simulink subsystem "H175_cathode"  (R2022b)
settings: Solver=VariableStepAuto  StartTime=0.0  StopTime=10.0  RelTol=1e-3
libraries: fl_lib x88, nesl_utility x73, SimscapeFluids_lib x10, slpidlib x2, BraytonCycle_lib x2
(part 4 of 4)

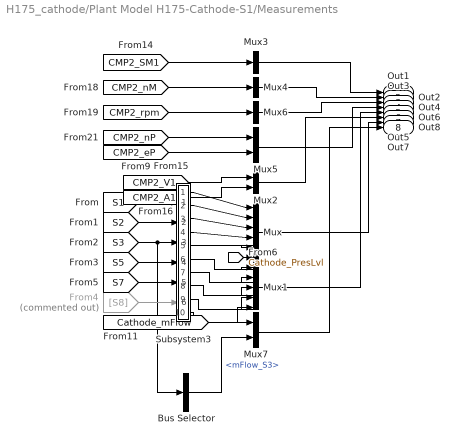
== system H175_cathode/Plant Model H175-Cathode-S1/Measurements ==
  Bus Selector : BusSelector  OutputSignals=mFlow_S3
  From4 : From  Commented=on  GotoTag=S8
  Mux : Mux  Inputs=6
  Mux1 : Mux  Inputs=5
  Mux2 : Mux  Inputs=2
  Mux3 : Mux  Inputs=1
  Mux4 : Mux  Inputs=1
  Mux5 : Mux  Inputs=2
  Mux6 : Mux  Inputs=1
  Mux7 : Mux  Inputs=2
  Subsystem3 : Subsystem
  Out1 : Outport
  Out2 : Outport  Port=2
  Out3 : Outport  Port=3
  Out4 : Outport  Port=4
  Out5 : Outport  Port=5
  Out6 : Outport  Port=6
  Out7 : Outport  Port=7
  Out8 : Outport  Port=8
  wires:
  Mux4/1 -> Out2/1
  Mux6/1 -> Out3/1
  Mux/1 -> Out7/1
  Subsystem3/6(<aTemp_S1>) -> Mux1/1
  Subsystem3/4(<aPres_S5>) -> Mux/4
  [CMP2_rpm] -> Mux6/1
  Subsystem3/3(<aPres_S3>) -> Mux/3
  Subsystem3/9(<aTemp_S5>) -> Mux1/4
  [S3] -> Subsystem3/3(In5), Bus Selector/1
  Subsystem3/8(<aTemp_S3>) -> Mux1/3
  Subsystem3/5(<aPres_S7>) -> Mux/5
  [S5] -> Subsystem3/4(In6)
  [CMP2_nP] -> Mux5/1
  Mux1/1 -> Out5/1
  Subsystem3/2(<aPres_S2>) -> Mux/2
  Mux7/1 -> Out8/1
  [CMP2_V1] -> Mux2/1
  From4/1 -> Subsystem3/6(In8)
  [S2] -> Subsystem3/2(In4)
  [CMP2_nM] -> Mux4/1
  Subsystem3/1(<aPres_S1>) -> Mux/1
  Bus Selector/1 -> Mux7/2  "<mFlow_S3>"
  Mux5/1 -> Out4/1
  Mux2/1 -> Out6/1
  [CMP2_A1] -> Mux2/2
  [CMP2_SM1] -> Mux3/1
  Subsystem3/7(<aTemp_S2>) -> Mux1/2
  Subsystem3/10(<aTemp_S7>) -> Mux1/5
  [S7] -> Subsystem3/5(In7)
  [Cathode_mFlow] -> Mux7/1
  [CMP2_eP] -> Mux5/2
  Mux3/1 -> Out1/1
  [S1] -> Subsystem3/1(In3)
  [Cathode_PresLvl] -> Mux/6

== system H175_cathode/Plant Model H175-Cathode-S1/Outlet ==
  Controlled Reservoir (G)1 : fl_lib/Gas/Elements/Controlled Reservoir (G)  area_A=0.002 m^2
      settings: InternalSimscapePortConfiguration="{\"Bottom\":[],\"Left\":[{\"id\":\"A\",\"label\":\"A\",\"type\":\"foundation.gas.gas\"}],\"Right\":[{\"id\":\"T_in\",\"label\":\"T\",\"type\":\"input\"},{\"id\":\"p_in\",\"label\":\"P\",\"type\":\"input\"}],\"Top\":[]}"
  Flow Resistance (G) : fl_lib/Gas/Elements/Flow Resistance (G)  delta_p_nominal=.15 bar  mdot_nominal=.3 kg/s  rho_nominal=2.1 kg/m^3  area=0.01 m^2  laminar_fraction=1e-3
      settings: InternalSimscapePortConfiguration="{\"Bottom\":[],\"Left\":[{\"id\":\"A\",\"label\":\"A\",\"type\":\"foundation.gas.gas\"}],\"Right\":[{\"id\":\"B\",\"label\":\"B\",\"type\":\"foundation.gas.gas\"}],\"Top\":[]}"
  Conn1 : PMIOPort  Side=Left
  Conn2 : PMIOPort  Port=2  Side=Left
  Conn3 : PMIOPort  Port=3  Side=Right
  connections:
  Flow Resistance (G)/RConn1 -- Conn3/RConn1
  Controlled Reservoir (G)1/RConn1 -- Conn2/RConn1
  Controlled Reservoir (G)1/LConn1 -- Flow Resistance (G)/LConn1
  Controlled Reservoir (G)1/RConn2 -- Conn1/RConn1

== system H175_cathode/Plant Model H175-Cathode-S1/S1 ==
  Absolute Reference (G) : fl_lib/Gas/Elements/Absolute Reference (G)
      settings: InternalSimscapePortConfiguration="{\"Bottom\":[],\"Left\":[{\"id\":\"A\",\"label\":\"\",\"type\":\"foundation.gas.gas\"}],\"Right\":[],\"Top\":[]}"
  Bus Creator : BusCreator  Inputs=3
  Mass & Energy Flow Rate Sensor (G) : fl_lib/Gas/Sensors/Mass & Energy Flow Rate Sensor (G)
      settings: InternalSimscapePortConfiguration="{\"Bottom\":[],\"Left\":[{\"id\":\"A\",\"label\":\"A\",\"type\":\"foundation.gas.gas\"}],\"Right\":[{\"id\":\"B\",\"label\":\"B\",\"type\":\"foundation.gas.gas\"},{\"id\":\"M\",\"label\":\"M\",\"type\":\"output\"},{\"id\":\"PHI\",\"label\":\"Phi\",\"type\":\"output\"}],\"Top\":[]}"
  Pressure & Temperature Sensor (G)4 : fl_lib/Gas/Sensors/Pressure & Temperature Sensor (G)
      settings: InternalSimscapePortConfiguration="{\"Bottom\":[],\"Left\":[{\"id\":\"A\",\"label\":\"A\",\"type\":\"foundation.gas.gas\"}],\"Right\":[{\"id\":\"B\",\"label\":\"B\",\"type\":\"foundation.gas.gas\"},{\"id\":\"P\",\"label\":\"P\",\"type\":\"output\"},{\"id\":\"T\",\"label\":\"T\",\"type\":\"output\"}],\"Top\":[]}"
  aPres_S1 : nesl_utility/PS-Simulink Converter  PhysicalDomain=network_engine_domain  SubClassName=ps_output  LeftPortType=input  RightPortType=output  PseudoPeriodic=off  Frequencies=[]  VectorFormat=inherit  Unit=inherit  AffineConversion=off
  aTemp_S1 : nesl_utility/PS-Simulink Converter  PhysicalDomain=network_engine_domain  SubClassName=ps_output  LeftPortType=input  RightPortType=output  PseudoPeriodic=off  Frequencies=[]  VectorFormat=inherit  Unit=inherit  AffineConversion=off
  aTemp_S2 : nesl_utility/PS-Simulink Converter  PhysicalDomain=network_engine_domain  SubClassName=ps_output  LeftPortType=input  RightPortType=output  PseudoPeriodic=off  Frequencies=[]  VectorFormat=inherit  Unit=inherit  AffineConversion=off
  Conn1 : PMIOPort  Side=Left
  Conn2 : PMIOPort  Port=2  Side=Right
  Out1 : Outport
  wires:
  aTemp_S2/1 -> Bus Creator/3  "mFlow_S1"
  Bus Creator/1 -> Out1/1
  aPres_S1/1 -> Bus Creator/1  "aPres_S1"
  aTemp_S1/1 -> Bus Creator/2  "aTemp_S1"
  connections:
  Mass & Energy Flow Rate Sensor (G)/RConn1 -- Conn2/RConn1
  Mass & Energy Flow Rate Sensor (G)/RConn2 -- aTemp_S2/LConn1
  Conn1/RConn1 -- Pressure & Temperature Sensor (G)4/LConn1 -- Mass & Energy Flow Rate Sensor (G)/LConn1
  aTemp_S1/LConn1 -- Pressure & Temperature Sensor (G)4/RConn3
  aPres_S1/LConn1 -- Pressure & Temperature Sensor (G)4/RConn2
  Absolute Reference (G)/LConn1 -- Pressure & Temperature Sensor (G)4/RConn1

== system H175_cathode/Plant Model H175-Cathode-S1/S2 ==
  Absolute Reference (G) : fl_lib/Gas/Elements/Absolute Reference (G)
      settings: InternalSimscapePortConfiguration="{\"Bottom\":[],\"Left\":[{\"id\":\"A\",\"label\":\"\",\"type\":\"foundation.gas.gas\"}],\"Right\":[],\"Top\":[]}"
  Bus Creator : BusCreator  Inputs=3
  Mass & Energy Flow Rate Sensor (G) : fl_lib/Gas/Sensors/Mass & Energy Flow Rate Sensor (G)
      settings: InternalSimscapePortConfiguration="{\"Bottom\":[],\"Left\":[{\"id\":\"A\",\"label\":\"A\",\"type\":\"foundation.gas.gas\"}],\"Right\":[{\"id\":\"B\",\"label\":\"B\",\"type\":\"foundation.gas.gas\"},{\"id\":\"M\",\"label\":\"M\",\"type\":\"output\"},{\"id\":\"PHI\",\"label\":\"Phi\",\"type\":\"output\"}],\"Top\":[]}"
  Pressure & Temperature Sensor (G)4 : fl_lib/Gas/Sensors/Pressure & Temperature Sensor (G)
      settings: InternalSimscapePortConfiguration="{\"Bottom\":[],\"Left\":[{\"id\":\"A\",\"label\":\"A\",\"type\":\"foundation.gas.gas\"}],\"Right\":[{\"id\":\"B\",\"label\":\"B\",\"type\":\"foundation.gas.gas\"},{\"id\":\"P\",\"label\":\"P\",\"type\":\"output\"},{\"id\":\"T\",\"label\":\"T\",\"type\":\"output\"}],\"Top\":[]}"
  aPres_S1 : nesl_utility/PS-Simulink Converter  PhysicalDomain=network_engine_domain  SubClassName=ps_output  LeftPortType=input  RightPortType=output  PseudoPeriodic=off  Frequencies=[]  VectorFormat=inherit  Unit=inherit  AffineConversion=off
  aTemp_S1 : nesl_utility/PS-Simulink Converter  PhysicalDomain=network_engine_domain  SubClassName=ps_output  LeftPortType=input  RightPortType=output  PseudoPeriodic=off  Frequencies=[]  VectorFormat=inherit  Unit=degC  AffineConversion=off
  mFlow_S2 : nesl_utility/PS-Simulink Converter  PhysicalDomain=network_engine_domain  SubClassName=ps_output  LeftPortType=input  RightPortType=output  PseudoPeriodic=off  Frequencies=[]  VectorFormat=inherit  Unit=inherit  AffineConversion=off
  Conn1 : PMIOPort  Side=Left
  Conn2 : PMIOPort  Port=2  Side=Right
  Out1 : Outport
  wires:
  mFlow_S2/1 -> Bus Creator/3  "mFlow_S2"
  aTemp_S1/1 -> Bus Creator/2  "aTemp_S2"
  aPres_S1/1 -> Bus Creator/1  "aPres_S2"
  Bus Creator/1 -> Out1/1
  connections:
  Mass & Energy Flow Rate Sensor (G)/RConn2 -- mFlow_S2/LConn1
  Mass & Energy Flow Rate Sensor (G)/RConn1 -- Conn2/RConn1
  aTemp_S1/LConn1 -- Pressure & Temperature Sensor (G)4/RConn3
  aPres_S1/LConn1 -- Pressure & Temperature Sensor (G)4/RConn2
  Absolute Reference (G)/LConn1 -- Pressure & Temperature Sensor (G)4/RConn1
  Conn1/RConn1 -- Mass & Energy Flow Rate Sensor (G)/LConn1 -- Pressure & Temperature Sensor (G)4/LConn1

== system H175_cathode/Plant Model H175-Cathode-S1/S3 ==
  Absolute Reference (G) : fl_lib/Gas/Elements/Absolute Reference (G)
      settings: InternalSimscapePortConfiguration="{\"Bottom\":[],\"Left\":[{\"id\":\"A\",\"label\":\"\",\"type\":\"foundation.gas.gas\"}],\"Right\":[],\"Top\":[]}"
  Bus Creator : BusCreator  Inputs=3
  Mass & Energy Flow Rate Sensor (G) : fl_lib/Gas/Sensors/Mass & Energy Flow Rate Sensor (G)
      settings: InternalSimscapePortConfiguration="{\"Bottom\":[],\"Left\":[{\"id\":\"A\",\"label\":\"A\",\"type\":\"foundation.gas.gas\"}],\"Right\":[{\"id\":\"B\",\"label\":\"B\",\"type\":\"foundation.gas.gas\"},{\"id\":\"M\",\"label\":\"M\",\"type\":\"output\"},{\"id\":\"PHI\",\"label\":\"Phi\",\"type\":\"output\"}],\"Top\":[]}"
  Pressure & Temperature Sensor (G)4 : fl_lib/Gas/Sensors/Pressure & Temperature Sensor (G)
      settings: InternalSimscapePortConfiguration="{\"Bottom\":[],\"Left\":[{\"id\":\"A\",\"label\":\"A\",\"type\":\"foundation.gas.gas\"}],\"Right\":[{\"id\":\"B\",\"label\":\"B\",\"type\":\"foundation.gas.gas\"},{\"id\":\"P\",\"label\":\"P\",\"type\":\"output\"},{\"id\":\"T\",\"label\":\"T\",\"type\":\"output\"}],\"Top\":[]}"
  aPres_S1 : nesl_utility/PS-Simulink Converter  PhysicalDomain=network_engine_domain  SubClassName=ps_output  LeftPortType=input  RightPortType=output  PseudoPeriodic=off  Frequencies=[]  VectorFormat=inherit  Unit=inherit  AffineConversion=off
  aPres_S2 : nesl_utility/PS-Simulink Converter  PhysicalDomain=network_engine_domain  SubClassName=ps_output  LeftPortType=input  RightPortType=output  PseudoPeriodic=off  Frequencies=[]  VectorFormat=inherit  Unit=inherit  AffineConversion=off
  aTemp_S1 : nesl_utility/PS-Simulink Converter  PhysicalDomain=network_engine_domain  SubClassName=ps_output  LeftPortType=input  RightPortType=output  PseudoPeriodic=off  Frequencies=[]  VectorFormat=inherit  Unit=degC  AffineConversion=off
  Conn2 : PMIOPort  Side=Left
  Conn1 : PMIOPort  Port=2  Side=Right
  Out1 : Outport
  wires:
  aPres_S2/1 -> Bus Creator/3  "mFlow_S3"
  Bus Creator/1 -> Out1/1
  aPres_S1/1 -> Bus Creator/1  "aPres_S3"
  aTemp_S1/1 -> Bus Creator/2  "aTemp_S3"
  connections:
  Mass & Energy Flow Rate Sensor (G)/RConn2 -- aPres_S2/LConn1
  Conn1/RConn1 -- Mass & Energy Flow Rate Sensor (G)/LConn1 -- Pressure & Temperature Sensor (G)4/LConn1
  aTemp_S1/LConn1 -- Pressure & Temperature Sensor (G)4/RConn3
  aPres_S1/LConn1 -- Pressure & Temperature Sensor (G)4/RConn2
  Absolute Reference (G)/LConn1 -- Pressure & Temperature Sensor (G)4/RConn1
  Mass & Energy Flow Rate Sensor (G)/RConn1 -- Conn2/RConn1

== system H175_cathode/Plant Model H175-Cathode-S1/S5 ==
  Absolute Reference (G) : fl_lib/Gas/Elements/Absolute Reference (G)
      settings: InternalSimscapePortConfiguration="{\"Bottom\":[],\"Left\":[{\"id\":\"A\",\"label\":\"\",\"type\":\"foundation.gas.gas\"}],\"Right\":[],\"Top\":[]}"
  Bus Creator : BusCreator  Inputs=2
  Pressure & Temperature Sensor (G)4 : fl_lib/Gas/Sensors/Pressure & Temperature Sensor (G)
      settings: InternalSimscapePortConfiguration="{\"Bottom\":[],\"Left\":[{\"id\":\"A\",\"label\":\"A\",\"type\":\"foundation.gas.gas\"}],\"Right\":[{\"id\":\"B\",\"label\":\"B\",\"type\":\"foundation.gas.gas\"},{\"id\":\"P\",\"label\":\"P\",\"type\":\"output\"},{\"id\":\"T\",\"label\":\"T\",\"type\":\"output\"}],\"Top\":[]}"
  aPres_S1 : nesl_utility/PS-Simulink Converter  PhysicalDomain=network_engine_domain  SubClassName=ps_output  LeftPortType=input  RightPortType=output  PseudoPeriodic=off  Frequencies=[]  VectorFormat=inherit  Unit=inherit  AffineConversion=off
  aTemp_S1 : nesl_utility/PS-Simulink Converter  PhysicalDomain=network_engine_domain  SubClassName=ps_output  LeftPortType=input  RightPortType=output  PseudoPeriodic=off  Frequencies=[]  VectorFormat=inherit  Unit=degC  AffineConversion=off
  Conn1 : PMIOPort  Side=Left
  Conn2 : PMIOPort  Port=2  Side=Right
  Out1 : Outport
  wires:
  aTemp_S1/1 -> Bus Creator/2  "aTemp_S5"
  aPres_S1/1 -> Bus Creator/1  "aPres_S5"
  Bus Creator/1 -> Out1/1
  connections:
  aTemp_S1/LConn1 -- Pressure & Temperature Sensor (G)4/RConn3
  aPres_S1/LConn1 -- Pressure & Temperature Sensor (G)4/RConn2
  Absolute Reference (G)/LConn1 -- Pressure & Temperature Sensor (G)4/RConn1
  Conn2/RConn1 -- Conn1/RConn1 -- Pressure & Temperature Sensor (G)4/LConn1

== system H175_cathode/Plant Model H175-Cathode-S1/S7 ==
  Absolute Reference (G) : fl_lib/Gas/Elements/Absolute Reference (G)
      settings: InternalSimscapePortConfiguration="{\"Bottom\":[],\"Left\":[{\"id\":\"A\",\"label\":\"\",\"type\":\"foundation.gas.gas\"}],\"Right\":[],\"Top\":[]}"
  Bus Creator : BusCreator  Inputs=3
  Mass & Energy Flow Rate Sensor (G) : fl_lib/Gas/Sensors/Mass & Energy Flow Rate Sensor (G)
      settings: InternalSimscapePortConfiguration="{\"Bottom\":[],\"Left\":[{\"id\":\"A\",\"label\":\"A\",\"type\":\"foundation.gas.gas\"}],\"Right\":[{\"id\":\"B\",\"label\":\"B\",\"type\":\"foundation.gas.gas\"},{\"id\":\"M\",\"label\":\"M\",\"type\":\"output\"},{\"id\":\"PHI\",\"label\":\"Phi\",\"type\":\"output\"}],\"Top\":[]}"
  Pressure & Temperature Sensor (G)4 : fl_lib/Gas/Sensors/Pressure & Temperature Sensor (G)
      settings: InternalSimscapePortConfiguration="{\"Bottom\":[],\"Left\":[{\"id\":\"A\",\"label\":\"A\",\"type\":\"foundation.gas.gas\"}],\"Right\":[{\"id\":\"B\",\"label\":\"B\",\"type\":\"foundation.gas.gas\"},{\"id\":\"P\",\"label\":\"P\",\"type\":\"output\"},{\"id\":\"T\",\"label\":\"T\",\"type\":\"output\"}],\"Top\":[]}"
  aPres_S1 : nesl_utility/PS-Simulink Converter  PhysicalDomain=network_engine_domain  SubClassName=ps_output  LeftPortType=input  RightPortType=output  PseudoPeriodic=off  Frequencies=[]  VectorFormat=inherit  Unit=inherit  AffineConversion=off
  aTemp_S1 : nesl_utility/PS-Simulink Converter  PhysicalDomain=network_engine_domain  SubClassName=ps_output  LeftPortType=input  RightPortType=output  PseudoPeriodic=off  Frequencies=[]  VectorFormat=inherit  Unit=degC  AffineConversion=off
  mFlow_S7 : nesl_utility/PS-Simulink Converter  PhysicalDomain=network_engine_domain  SubClassName=ps_output  LeftPortType=input  RightPortType=output  PseudoPeriodic=off  Frequencies=[]  VectorFormat=inherit  Unit=kg/s  AffineConversion=off
  Conn1 : PMIOPort  Side=Left
  Conn2 : PMIOPort  Port=2  Side=Right
  Out1 : Outport
  wires:
  mFlow_S7/1 -> Bus Creator/3  "mFlow_S7"
  Bus Creator/1 -> Out1/1
  aPres_S1/1 -> Bus Creator/1  "aPres_S7"
  aTemp_S1/1 -> Bus Creator/2  "aTemp_S7"
  connections:
  Conn2/RConn1 -- Mass & Energy Flow Rate Sensor (G)/RConn1
  Mass & Energy Flow Rate Sensor (G)/RConn2 -- mFlow_S7/LConn1
  aTemp_S1/LConn1 -- Pressure & Temperature Sensor (G)4/RConn3
  aPres_S1/LConn1 -- Pressure & Temperature Sensor (G)4/RConn2
  Absolute Reference (G)/LConn1 -- Pressure & Temperature Sensor (G)4/RConn1
  Mass & Energy Flow Rate Sensor (G)/LConn1 -- Pressure & Temperature Sensor (G)4/LConn1 -- Conn1/RConn1

== system H175_cathode/Plant Model H175-Cathode-S1/Subsystem ==
  Bus Selector : BusSelector  OutputSignals=aPres_S1,aTemp_S1
  Bus Selector1 : BusSelector  OutputSignals=aPres_S2
  Bus Selector2 : BusSelector  OutputSignals=aTemp_S3,aPres_S3,mFlow_S3
  <aPres_S1> : Outport
  <aTemp_S1> : Outport  Port=2
  <mFlow_S2> : Outport  Port=3
  <aPres_S2> : Outport  Port=4
  <aTemp_S3> : Outport  Port=5
  <aPres_S3> : Outport  Port=6
  wires:
  Bus Selector2/3 -> <mFlow_S2>/1  "<mFlow_S3>"
  Bus Selector2/2 -> <aPres_S3>/1  "<aPres_S3>"
  Bus Selector/2 -> <aTemp_S1>/1  "<aTemp_S1>"
  Bus Selector1/1 -> <aPres_S2>/1  "<aPres_S2>"
  Bus Selector2/1 -> <aTemp_S3>/1  "<aTemp_S3>"
  [S3] -> Bus Selector2/1
  [S1] -> Bus Selector/1
  Bus Selector/1 -> <aPres_S1>/1  "<aPres_S1>"
  [S2] -> Bus Selector1/1

== system H175_cathode/Plant Model H175-Cathode-S1/VL6513 ==
  input0 : Inport
  Display : Display
  Orifice (G) : SimscapeFluids_lib/Gas/Valves & Orifices/Orifice (G)  orifice_type=foundation.enum.constant_variable.variable  orifice_parameterization=fluids.gas.valves_orifices.enum.OrificeParameterization.Area  opening_characteristic=fluids.gas.valves_orifices.enum.OpeningCharacteristics.Tabulated  Cv_constant=4  Cv_max=169.7  L_Cv_TLU=0 : 0.2 : 1  Cv_TLU=[1e-06, .8, 1.6, 2.4, 3.2, 4]  xT_Cv=0.7  Kv_constant=3.6  Kv_max=10  L_Kv_TLU=0 : 0.2 : 1  Kv_TLU=[1e-06, .72, 1.44, 2.16, 2.88, 3.6]  xT_Kv=0.7  C_constant=12 l/(bar*s)  B_crit_constant=0.3  C_max=12 l/(bar*s)  B_crit_linear=0.3  L_C_TLU=0 : 0.2 : 1  C_TLU=[1e-05, 2.4, 4.8, 7.2, 9.6, 12] l/(bar*s)  B_crit_TLU=0.3 * ones(1, 6)  m=0.5  T_ref_C=293.15 K  rho_ref_C=1.185 kg/m^3  orifice_area_constant=1e-4 m^2  orifice_area_max=0.00145 m^2  L_orifice_area_TLU=[0.00889,0.15555,0.26,0.36444,0.46889,0.57222,0.676666,0.7811,0.88555,0.9277]  orifice_area_TLU=[0.000258,0.00146,0.001674,0.0018,0.00189,0.001946,0.0019564,0.001995,0.001999,0.002] m^2  Cd=.8  leakage_fraction=1e-6  smoothing_factor=0.02  B_lam=0.999  area=0.0021 m^2  mdot_A_specify=off  mdot_A_priority=None  mdot_A=0 kg/s  mdot_A_nominal_specify=off  mdot_A_nominal_unit=kg/s  mdot_A_nominal_value=1  mdot_B_specify=off  mdot_B_priority=None  mdot_B=0 kg/s  mdot_B_nominal_specify=off  mdot_B_nominal_unit=kg/s  mdot_B_nominal_value=1  Phi_A_specify=off  Phi_A_priority=None  Phi_A=0 kW  Phi_A_nominal_specify=off  Phi_A_nominal_unit=kW  Phi_A_nominal_value=1  Phi_B_specify=off  Phi_B_priority=None  Phi_B=0 kW  Phi_B_nominal_specify=off  Phi_B_nominal_unit=kW  Phi_B_nominal_value=1
      settings: InternalSimscapePortConfiguration="{\"Bottom\":[],\"Left\":[{\"id\":\"A\",\"label\":\"A\",\"type\":\"foundation.gas.gas\"},{\"id\":\"L\",\"label\":\"L\",\"type\":\"input\"}],\"Right\":[{\"id\":\"B\",\"label\":\"B\",\"type\":\"foundation.gas.gas\"}],\"Top\":[]}"
  Simulink-PS Converter3 : nesl_utility/Simulink-PS Converter  PhysicalDomain=network_engine_domain  SubClassName=ps_input  LeftPortType=input  RightPortType=output  PseudoPeriodic=off  Frequencies=[]  NoiseDistribution=none  NoiseParameters=[]  Unit=1  AffineConversion=off  FilteringAndDerivatives=filter  SimscapeFilterOrder=1  InputFilterTimeConstant=0.001  UdotUserProvided=0
  Conn1 : PMIOPort  Side=Left
  Conn2 : PMIOPort  Port=2  Side=Right
  wires:
  input0/1 -> Simulink-PS Converter3/1, Display/1
  connections:
  Orifice (G)/LConn1 -- Conn2/RConn1
  Conn1/RConn1 -- Orifice (G)/RConn1
  Simulink-PS Converter3/RConn1 -- Orifice (G)/LConn2

== system H175_cathode/Humidifier/Cathode Humidifier1/Proportional Control ==
  RH_set : Inport
  RH_meas : Inport  Port=2
  Gain : Gain  Commented=on  Gain=0.1
  PID Controller : slpidlib/PID Controller  Controller=PI  Form=Parallel  TimeDomain=Continuous-time  UseExternalTs=off  SampleTime=-1  IntegratorMethod=Forward Euler  FilterMethod=Forward Euler  ControllerParametersSource=internal  P=1  I=1  UseKiTs=off  D=0  N=100  UseFilter=on  TunerSelectOption=Transfer Function Based (PID Tuner App)  InitialConditionSource=internal  InitialConditionForIntegrator=0  InitialConditionForFilter=0  DifferentiatorICPrevScaledInput=0  ExternalReset=none  TrackingMode=off  Kt=1  LimitOutput=off  SatLimitsSource=internal  UpperSaturationLimit=inf  LowerSaturationLimit=-inf  LinearizeAsGain=on  AntiWindupMode=none  Kb=1  LimitIntegrator=off  UpperIntegratorSaturationLimit=inf  LowerIntegratorSaturationLimit=-inf  POutMin=[]  POutMax=[]  IOutMin=[]  IOutMax=[]  DOutMin=[]  DOutMax=[]  NOutMin=[]  NOutMax=[]  SumOutMin=[]  SumOutMax=[]  SaturationOutMin=[]  SaturationOutMax=[]  PParamMin=[]  PParamMax=[]  IParamMin=[]  IParamMax=[]  DParamMin=[]  DParamMax=[]  NParamMin=[]  NParamMax=[]  KbParamMin=[]  KbParamMax=[]  KtParamMin=[]  KtParamMax=[]  KbOutMin=[]  KbOutMax=[]  KtOutMin=[]  KtOutMax=[]  IntegratorOutMin=[]  IntegratorOutMax=[]  FilterOutMin=[]  FilterOutMax=[]  SumI1OutMin=[]  SumI1OutMax=[]  SumI2OutMin=[]  SumI2OutMax=[]  SumI3OutMin=[]  SumI3OutMax=[]  SumI4OutMin=[]  SumI4OutMax=[]  SumDOutMin=[]  SumDOutMax=[]  DifferentiatorOutMin=[]  DifferentiatorOutMax=[]  FilterDiffOutCoefMin=[]  FilterDiffOutCoefMax=[]  ReciprocalOutMin=[]  ReciprocalOutMax=[]  SumDenOutMin=[]  SumDenOutMax=[]  SumNumOutMin=[]  SumNumOutMax=[]  DivideOutMin=[]  DivideOutMax=[]  UdiffTsProdOutMin=[]  UdiffTsProdOutMax=[]  NTsProdOutMin=[]  NTsProdOutMax=[]  UintegralTsProdOutMin=[]  UintegralTsProdOutMax=[]  UngainTsProdOutMin=[]  UngainTsProdOutMax=[]  ClampingZeroOutDataTypeStr=Inherit: Inherit via back propagation  ClampingZeroOutMin=[]  ClampingZeroOutMax=[]  FilterDenConstantOutDataTypeStr=Inherit: Inherit via back propagation  FilterDenConstantOutMin=[]  FilterDenConstantOutMax=[]  PCopyOutDataTypeStr=Inherit: Inherit via back propagation  PCopyOutMin=[]  PCopyOutMax=[]  NCopyOutDataTypeStr=Inherit: Inherit via back propagation  NCopyOutMin=[]  NCopyOutMax=[]  IntegratorContinuousStateAttributes=''  IntegratorStateMustResolveToSignalObject=off  IntegratorRTWStateStorageClass=Auto  FilterContinuousStateAttributes=''  FilterStateMustResolveToSignalObject=off  FilterRTWStateStorageClass=Auto  ParallelPVariant=InternalParameters  IdealPVariant=Disabled  IVariant=InternalParameters  DVariant=Disabled  IntegratorVariant=Continuous  SatVariant=Disabled  AWVariant=Passthrough  PCopyVariant=Disabled  TRVariant=Disabled  FdbkBlocksVariant=Forward  IdealPFdbkVariant=Disabled  SatFdbkVariant=Disabled  DerivativeFilterVariant=Disabled  NVariant=Disabled  NCopyVariant=Disabled_SignalSpec  FilterICVariant=Disabled  IntegratorICVariant=InternalICs  ExternalResetVariant=Disabled  TRSumVariant=Passthrough  SumFdbkVariant=Disabled  SumVariant=Sum_PI  TsampFilterVariant=InternalTs  TsampNgainVariant=Passthrough  TsampIntegralVariant=Passthrough  ExternalSaturationOutDataTypeStr=Inherit: Same as second input
  Saturation : Saturate  Commented=on  UpperLimit=inf  LowerLimit=0  ZeroCross=off
  Sum : Sum  Inputs=|+-
  Transfer Fcn : TransferFcn  Denominator=[1 1]
  Mw : Outport
  wires:
  PID Controller/1 -> Transfer Fcn/1
  Gain/1 -> Saturation/1
  Transfer Fcn/1 -> Mw/1
  RH_meas/1 -> Sum/2
  Sum/1 -> PID Controller/1
  RH_set/1 -> Sum/1

== system H175_cathode/Humidifier/Cathode Humidifier2/Proportional Control ==
  RH_set : Inport
  RH_meas : Inport  Port=2
  Gain : Gain  Gain=0.15
  Saturation : Saturate  UpperLimit=inf  LowerLimit=0  ZeroCross=off
  Sum : Sum  Inputs=|+-
  Transfer Fcn : TransferFcn  Denominator=[1 1]
  Mw : Outport
  wires:
  RH_set/1 -> Sum/1
  Sum/1 -> Gain/1
  RH_meas/1 -> Sum/2
  Transfer Fcn/1 -> Mw/1
  Gain/1 -> Saturation/1
  Saturation/1 -> Transfer Fcn/1

== system H175_cathode/Plant Model H175-Cathode-S1/  INTER6511/Coolant Tank1 ==
  Coolant Volume : fl_lib/Thermal Liquid/Elements/Translational Mechanical Converter (TL)  mech_orientation=foundation.enum.MechOrientationTranslational.Positive  displacement_spec=foundation.enum.DisplacementSpec.Calculate  x0=x_init m  interface_area=A m^2  dead_volume=A * 0.001 m^3  environment_spec=foundation.enum.pressure_spec.atmospheric  environment_pressure=0.101325 MPa  dynamic_compressibility=simscape.enum.onoff.off  p0=env_p MPa  T0=20 degC
      settings: InternalSimscapePortConfiguration="{\"Bottom\":[],\"Left\":[{\"id\":\"A\",\"label\":\"A\",\"type\":\"foundation.thermal_liquid.thermal_liquid\"},{\"id\":\"C\",\"label\":\"C\",\"type\":\"foundation.mechanical.translational.translational\"},{\"id\":\"H\",\"label\":\"H\",\"type\":\"foundation.thermal.thermal\"}],\"Right\":[{\"id\":\"R\",\"label\":\"R\",\"type\":\"foundation.mechanical.translational.translational\"}],\"Top\":[]}"
  Mechanical Translational Reference : fl_lib/Mechanical/Translational Elements/Mechanical Translational Reference
  Perfect Insulator : fl_lib/Thermal/Thermal Elements/Perfect Insulator  T_specify=off  T_priority=None  T=0 K  T_nominal_specify=off  T_nominal_unit=K  T_nominal_value=1
  Translational Free End : fl_lib/Mechanical/Translational Elements/Translational Free End  v_specify=off  v_priority=None  v=0 m/s  v_nominal_specify=off  v_nominal_unit=m/s  v_nominal_value=1
      settings: InternalSimscapePortConfiguration="{\"Bottom\":[],\"Left\":[{\"id\":\"V\",\"label\":\"\",\"type\":\"foundation.mechanical.translational.translational\"}],\"Right\":[],\"Top\":[]}"
  T : PMIOPort  Side=Right
  connections:
  Perfect Insulator/LConn1 -- Coolant Volume/LConn3
  Translational Free End/LConn1 -- Coolant Volume/RConn1
  Mechanical Translational Reference/LConn1 -- Coolant Volume/LConn2
  Coolant Volume/LConn1 -- T/RConn1

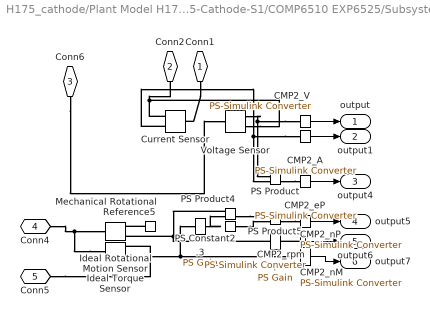
== system H175_cathode/Plant Model H175-Cathode-S1/COMP6510 EXP6525/Subsystem5 ==
  . : fl_lib/Physical Signals/Functions/PS Gain  gain=1/(0.1047198)
  .3 : fl_lib/Physical Signals/Functions/PS Gain  gain=1/(0.1047198*60)
  CMP2_A : nesl_utility/PS-Simulink Converter  PhysicalDomain=network_engine_domain  SubClassName=ps_output  LeftPortType=input  RightPortType=output  PseudoPeriodic=off  Frequencies=[]  VectorFormat=inherit  Unit=inherit  AffineConversion=off
  CMP2_V : nesl_utility/PS-Simulink Converter  PhysicalDomain=network_engine_domain  SubClassName=ps_output  LeftPortType=input  RightPortType=output  PseudoPeriodic=off  Frequencies=[]  VectorFormat=inherit  Unit=inherit  AffineConversion=off
  CMP2_eP : nesl_utility/PS-Simulink Converter  PhysicalDomain=network_engine_domain  SubClassName=ps_output  LeftPortType=input  RightPortType=output  PseudoPeriodic=off  Frequencies=[]  VectorFormat=inherit  Unit=inherit  AffineConversion=off
  CMP2_nM : nesl_utility/PS-Simulink Converter  PhysicalDomain=network_engine_domain  SubClassName=ps_output  LeftPortType=input  RightPortType=output  PseudoPeriodic=off  Frequencies=[]  VectorFormat=1-D array  Unit=inherit  AffineConversion=off
  CMP2_nP : nesl_utility/PS-Simulink Converter  PhysicalDomain=network_engine_domain  SubClassName=ps_output  LeftPortType=input  RightPortType=output  PseudoPeriodic=off  Frequencies=[]  VectorFormat=inherit  Unit=inherit  AffineConversion=off
  CMP2_rpm : nesl_utility/PS-Simulink Converter  PhysicalDomain=network_engine_domain  SubClassName=ps_output  LeftPortType=input  RightPortType=output  PseudoPeriodic=off  Frequencies=[]  VectorFormat=inherit  Unit=inherit  AffineConversion=off
  Current Sensor : fl_lib/Electrical/Electrical Sensors/Current Sensor
  Ideal Rotational Motion Sensor : fl_lib/Mechanical/Mechanical Sensors/Ideal Rotational Motion Sensor  reference=foundation.enum.MeasurementReference.difference  acceleration_port=false  velocity_port=true  position_port=false  wrap_angle=false  offset=0 rad
      settings: InternalSimscapePortConfiguration="{\"Bottom\":[],\"Left\":[{\"id\":\"R\",\"label\":\"R\",\"type\":\"foundation.mechanical.rotational.rotational\"}],\"Right\":[{\"id\":\"C\",\"label\":\"C\",\"type\":\"foundation.mechanical.rotational.rotational\"},{\"id\":\"W\",\"label\":\"W\",\"type\":\"output\"}],\"Top\":[]}"
  Ideal Torque Sensor : fl_lib/Mechanical/Mechanical Sensors/Ideal Torque Sensor
      settings: LogSimulationData=on
  Mechanical Rotational Reference5 : fl_lib/Mechanical/Rotational Elements/Mechanical Rotational Reference
  PS Constant2 : fl_lib/Physical Signals/Sources/PS Constant  constant=2*pi
  PS Product : fl_lib/Physical Signals/Functions/PS Product
  PS Product4 : fl_lib/Physical Signals/Functions/PS Product
  PS Product5 : fl_lib/Physical Signals/Functions/PS Product
  Voltage Sensor : fl_lib/Electrical/Electrical Sensors/Voltage Sensor
  Conn1 : PMIOPort  Side=Left
  Conn2 : PMIOPort  Port=2  Side=Left
  Conn6 : PMIOPort  Port=3  Side=Left
  Conn4 : PMIOPort  Port=4  Side=Left
  Conn5 : PMIOPort  Port=5  Side=Left
  output : Outport
  output1 : Outport  Port=2
  output4 : Outport  Port=3
  output5 : Outport  Port=4
  output6 : Outport  Port=5
  output7 : Outport  Port=6
  wires:
  CMP2_A/1 -> output1/1
  CMP2_nP/1 -> output5/1
  CMP2_V/1 -> output/1
  CMP2_nM/1 -> output7/1
  CMP2_eP/1 -> output4/1
  CMP2_rpm/1 -> output6/1
  connections:
  Conn6/RConn1 -- Voltage Sensor/LConn1
  Conn2/RConn1 -- Voltage Sensor/RConn2 -- Current Sensor/RConn2
  PS Product4/RConn1 -- PS Product5/LConn1
  PS Constant2/RConn1 -- PS Product5/LConn2
  Conn1/RConn1 -- Current Sensor/LConn1
  Ideal Torque Sensor/LConn1 -- Ideal Rotational Motion Sensor/LConn1 -- Conn4/RConn1
  .3/LConn1 -- CMP2_nM/LConn1 -- Ideal Torque Sensor/RConn2
  PS Product5/RConn1 -- CMP2_nP/LConn1
  CMP2_V/LConn1 -- PS Product/LConn2 -- Voltage Sensor/RConn1
  PS Product/RConn1 -- CMP2_eP/LConn1
  .3/RConn1 -- PS Product4/LConn2
  CMP2_rpm/LConn1 -- ./RConn1
  CMP2_A/LConn1 -- PS Product/LConn1 -- Current Sensor/RConn1
  Ideal Rotational Motion Sensor/RConn2 -- PS Product4/LConn1 -- ./LConn1
  Mechanical Rotational Reference5/LConn1 -- Ideal Rotational Motion Sensor/RConn1
  Conn5/RConn1 -- Ideal Torque Sensor/RConn1

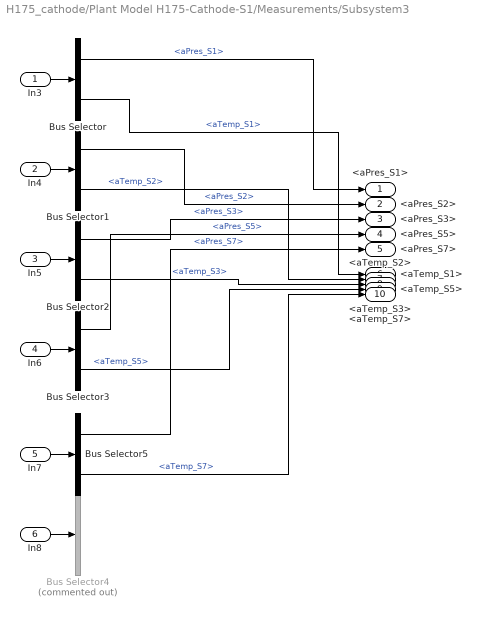
== system H175_cathode/Plant Model H175-Cathode-S1/Measurements/Subsystem3 ==
  In3 : Inport
  In4 : Inport  Port=2
  In5 : Inport  Port=3
  In6 : Inport  Port=4
  In7 : Inport  Port=5
  In8 : Inport  Port=6
  Bus Selector : BusSelector  OutputSignals=aPres_S1,aTemp_S1
  Bus Selector1 : BusSelector  OutputSignals=aPres_S2,aTemp_S2
  Bus Selector2 : BusSelector  OutputSignals=aPres_S3,aTemp_S3
  Bus Selector3 : BusSelector  OutputSignals=aPres_S5,aTemp_S5
  Bus Selector4 : BusSelector  Commented=on  OutputSignals=aPres_S8,aTemp_S8,mFlow_S8,MixSEnthalpy_S8,MixDensity_S8,SHeat_S8,SEntropy_S8
  Bus Selector5 : BusSelector  OutputSignals=aPres_S7,aTemp_S7
  <aPres_S1> : Outport
  <aPres_S2> : Outport  Port=2
  <aPres_S3> : Outport  Port=3
  <aPres_S5> : Outport  Port=4
  <aPres_S7> : Outport  Port=5
  <aTemp_S1> : Outport  Port=6
  <aTemp_S2> : Outport  Port=7
  <aTemp_S3> : Outport  Port=8
  <aTemp_S5> : Outport  Port=9
  <aTemp_S7> : Outport  Port=10
  wires:
  In6/1 -> Bus Selector3/1
  Bus Selector3/1 -> <aPres_S5>/1  "<aPres_S5>"
  Bus Selector/1 -> <aPres_S1>/1  "<aPres_S1>"
  Bus Selector1/1 -> <aPres_S2>/1  "<aPres_S2>"
  Bus Selector/2 -> <aTemp_S1>/1  "<aTemp_S1>"
  In7/1 -> Bus Selector5/1
  Bus Selector2/1 -> <aPres_S3>/1  "<aPres_S3>"
  Bus Selector5/2 -> <aTemp_S7>/1  "<aTemp_S7>"
  In5/1 -> Bus Selector2/1
  Bus Selector5/1 -> <aPres_S7>/1  "<aPres_S7>"
  Bus Selector3/2 -> <aTemp_S5>/1  "<aTemp_S5>"
  Bus Selector2/2 -> <aTemp_S3>/1  "<aTemp_S3>"
  In3/1 -> Bus Selector/1
  In8/1 -> Bus Selector4/1
  Bus Selector1/2 -> <aTemp_S2>/1  "<aTemp_S2>"
  In4/1 -> Bus Selector1/1
